simulink subsystem "Controller"  (R2021b)
settings: Solver=VariableStepAuto  StartTime=0.0  StopTime=10.0  RelTol=1e-3
libraries: simulink_extras x1
settings Model: Creator=vojtech.voska  LastModifiedBy=vojtech.voska

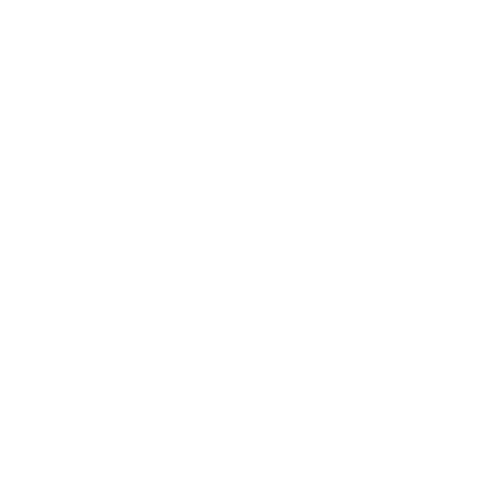
[thumbnail: Simulink's stored preview of the top-level diagram]
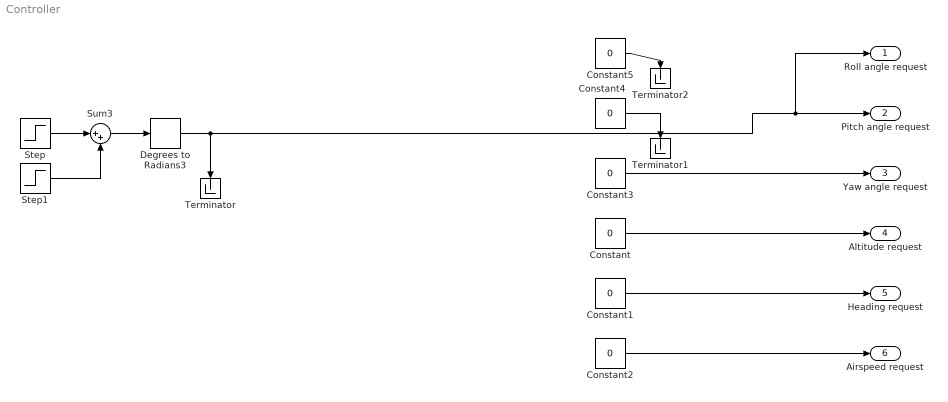
== system Controller ==
  Constant{,1..5} (6 alike) : Constant  Value=0
  Degrees to Radians3 : simulink_extras/Transformations/Degrees to Radians
  Step : Step  Time=5  After=5  SampleTime=0
  Step1 : Step  Time=15  After=-5  SampleTime=0
  Sum3 : Sum  Inputs=|++
  Terminator : Terminator
  Terminator1 : Terminator
  Terminator2 : Terminator
  Roll angle request : Outport  Unit=rad
  Pitch angle request : Outport  Port=2  Unit=rad
  Yaw angle request : Outport  Port=3  Unit=rad
  Altitude request : Outport  Port=4  Unit=rad
  Heading request : Outport  Port=5  Unit=rad
  Airspeed request : Outport  Port=6  Unit=rad
  wires:
  Step1/1 -> Sum3/2
  Step/1 -> Sum3/1
  Sum3/1 -> Degrees to Radians3/1
  Constant1/1 -> Heading request/1
  Constant2/1 -> Airspeed request/1
  Constant/1 -> Altitude request/1
  Constant3/1 -> Yaw angle request/1
  Degrees to Radians3/1 -> Terminator/1, Pitch angle request/1, Roll angle request/1
  Constant4/1 -> Terminator1/1
  Constant5/1 -> Terminator2/1
